simulink model "H250HILCtrl_400HzTypeXLOEUnknown"  (R2020b)
settings: Solver=FixedStepDiscrete  StartTime=0.0  StopTime=inf  FixedStep=Ts  RelTol=1e-3
InitFcn:
  | H250HILConInit_400HzTypeXLOEUnknown
values from neighbouring files (symbols this model uses):
  B = [0.25   -1.4142/(4*l)     1.4142/(4*l)     1/(4*c) ... (first row only)    [H250HILConInit_400HzTypeXLOEUnknown.m]
  g = (9.8)    (= 9.8)    [H250HILConInit_400HzTypeXLOEUnknown.m]
  J = (diag([0.0056 0.0056 0.0104]))    [H250HILConInit_400HzTypeXLOEUnknown.m]
  m = (0.752)    (= 0.752)    [H250HILConInit_400HzTypeXLOEUnknown.m]
  M = ([ 1          1          1         1 ... (first row only)    [H250HILConInit_400HzTypeXLOEUnknown.m]
  MY_ATT_P = Pixhawk_CSC.Parameter( {single(8), 'MY_ATT_P'}  )    [H250HILConInit_400HzTypeXLOEUnknown.m]
  MY_ATT_P_YAW = Pixhawk_CSC.Parameter( {single(0.0), 'MY_ATT_P_YAW'}  )    [H250HILConInit_400HzTypeXLOEUnknown.m]
  MY_POS_P = Pixhawk_CSC.Parameter( {single(0.6), 'MY_POS_P'}  )    [H250HILConInit_400HzTypeXLOEUnknown.m]
  MY_RATE_P = Pixhawk_CSC.Parameter( {single(12), 'MY_RATE_P'}  )    [H250HILConInit_400HzTypeXLOEUnknown.m]
  MY_RATE_P_YAW = Pixhawk_CSC.Parameter( {single(0.0), 'MY_RATE_P_YAW'}  )    [H250HILConInit_400HzTypeXLOEUnknown.m]
  MY_SAT_AD = Pixhawk_CSC.Parameter({single(0.13), 'MY_SAT_AD'} )    [H250HILConInit_400HzTypeXLOEUnknown.m]
  MY_TAU_P_A = Pixhawk_CSC.Parameter( {single(0.2), 'MY_TAU_P_A'}  )    [H250HILConInit_400HzTypeXLOEUnknown.m]
  MY_TAU_P_A_YAW = Pixhawk_CSC.Parameter( {single(0), 'MY_TAU_P_A_YAW'}  )    [H250HILConInit_400HzTypeXLOEUnknown.m]
  MY_TAU_P_P = Pixhawk_CSC.Parameter( {single(2.0), 'MY_TAU_P_P'}  )    [H250HILConInit_400HzTypeXLOEUnknown.m]
  MY_TAU_P_P_YAW = Pixhawk_CSC.Parameter( {single(0.04), 'MY_TAU_P_P_YAW'}  )    [H250HILConInit_400HzTypeXLOEUnknown.m]
  MY_VEL_P = Pixhawk_CSC.Parameter( {single(0.8), 'MY_VEL_P'}  )    [H250HILConInit_400HzTypeXLOEUnknown.m]
  T00 = single([m*g/4 m*g/4 m*g/4 m*g/4]')    [H250HILConInit_400HzTypeXLOEUnknown.m]
  Tf = 0.06    [H250HILConInit_400HzTypeXLOEUnknown.m]
  Tmotorbar = (0.032)    (= 0.032)    [H250HILConInit_400HzTypeXLOEUnknown.m]
  Ts = 1/400    (= 0.0025)    [H250HILConInit_400HzTypeXLOEUnknown.m]
libraries: discretizing x10, pixhawk_slib_uORB_RW x6, pixhawk_slib_sensors_actuators x5, pixhawk_slib_misc_utils x1, simulink x1, sharedtransform x1, pid_lib x1
(part 2 of 2)

== matlab function H250HILCtrl_400HzTypeXLOEUnknown/controller/innerloop/fmincon ==
  data: fd input; taop input; taoq input; taor input; T output; T0 input; M input; val output; time output
function [T,val,time] = fcn(fd, taop, taoq, taor, T0, M)
%% 求解
w1= 1;
w2 =20;
w3= 20;
w4= 0.00;
myfun2 = @(x)(w1*(M(1,:)*x-fd)^2+w2*(M(2,:)*x-taop)^2+w3*(M(3,:)*x-taoq)^2+w4*(M(4,:)*x-taor)^2);

lb  = [0 0 0 0]';
ub  = [3 3 3 3]';

options = optimoptions(@fmincon,'Algorithm','sqp','MaxIterations',10);
% tic
[T,val] = fmincon(myfun2,T0,[],[],[],[],lb,ub,[],options);
% ff = toc;
time =0;

== matlab function H250HILCtrl_400HzTypeXLOEUnknown/controller/innerloop/quadprog ==
  data: fd input double; taop input double; taoq input double; taor input double; T output double; T0 input double; M input double; fval output double; ub input double; iter output
function [T,fval, iter] = fcn(fd, taop, taoq, taor, T0, M, ub)
%% 求解
vd = [fd; taop; taoq; taor];
W=diag([1 20 20 0.01]);
H = M'*W*M;
f = -(vd'*W*M)';
% Td = B*vd;
lb  = [0 0 0 0]';
% ub  = [12 12 12 12]';
% if (max(B*vd)>3)||(min(B*vd)<0)
    options = optimoptions(@quadprog,'Algorithm','active-set','MaxIterations',10);

    [T,fval,~,output] = quadprog(H, f, [], [], [], [], lb, ub, T0, options);
     iter = output.iterations;
% else
%     T = B*vd;
%     fval = 0;
% end

== matlab function H250HILCtrl_400HzTypeXLOEUnknown/controller/innerloop/MATLAB Function1 ==
  data: u input; y output
function y = fcn(u)
y=diag([u,1,1,1]);

== matlab function H250HILCtrl_400HzTypeXLOEUnknown/controller/innerloop/MATLAB Function2 ==
  data: dT input; ub output
function ub = fcn(dT)
dub = zeros(4,1);
dub(1) = dT(1) - dT(3);
dub(2) = dT(2) - dT(4);
dub(3) = dT(3) - dT(1);
dub(4) = dT(4) - dT(2);
% dub(1) = dT(1);
% dub(2) = dT(2);
% dub(3) = dT(3);
% dub(4) = dT(4);
ub = [5 5 5 5]' + 1.8*min([dub(1) dub(2) dub(3) dub(4)]',[0 0 0 0]');%1.8

== matlab function H250HILCtrl_400HzTypeXLOEUnknown/controller/InputConditioning/MATLAB Function ==
  data: u input; y output
function y = fcn(u)

 if(u>1550)
    y=u;
 else
     if(u<1450)
     y=u;
     else
         y=single(1500);
     end
 end

== matlab function H250HILCtrl_400HzTypeXLOEUnknown/controller/InputConditioning/MATLAB Function1 ==
  data: u input; y output
function y = fcn(u)

 if(u>1550)
    y=u;
 else
     if(u<1450)
     y=u;
     else
         y=single(1500);
     end
 end

== matlab function H250HILCtrl_400HzTypeXLOEUnknown/controller/InputConditioning/MATLAB Function2 ==
  data: u input; y output
function y = fcn(u)

 if(u>1550)
    y=u;
 else
     if(u<1450)
     y=u;
     else
         y=single(1500);
     end
 end

== matlab function H250HILCtrl_400HzTypeXLOEUnknown/controller/quat2eul ==
  data: q input single; dcm output single
function dcm  = quat2eul(q)
% Conversion from Quaternion to Euler angles based on the PX4 Firmware
% v1.6.5 release.
% 
% Quaternion -> DCM -> Euler Angles
% INPUT:
%   q: Quaternion vector of the format: (a + bi + cj + dk)
% OUTPUT:
%   [phi,theta,psi]: Euler angles in radians.
% 
 if norm(q)~=0
    a = q(1);
    b = q(2);
    c = q(3);
    d = q(4);

    aSq = a*a;
    bSq = b*b;
    cSq = c*c;
    dSq = d*d;

    d_pi2 = pi/2;

    % quaternion_to_dcm
    dcm00 = aSq + bSq - cSq - dSq;
    dcm01 = 2*(b*c - a*d);
    dcm02 = 2*(a*c + b*d);
    dcm10 = 2*(b*c + a*d);
    dcm11 = aSq - bSq + cSq - dSq;
    dcm12 = 2*(c*d - a*b);
    dcm20 = 2*(b*d - a*c);
    dcm21 = 2*(a*b + c*d);
    dcm22 = aSq - bSq - cSq + dSq;
    dcm=[dcm00 dcm01 dcm02;
              dcm10 dcm11 dcm12;
              dcm20 dcm21  dcm22];
 else
     dcm = single(eye(3,3));
 end
    % dcm_to_euler

== matlab function H250HILCtrl_400HzTypeXLOEUnknown/controller/innerloop/Att ==
  data: e input; w input; psi input; pqrd output; ATT_P input; ATT_P_SCALE input
function pqrd  = fcn(e, w, psi, ATT_P, ATT_P_SCALE)
%% 角度控制1
% h1 = n3(1);
% h2 = n3(2);
% h3 = n3(3);
% h1d = n3d(1);
% h2d = n3d(2);
% h3d = n3d(3);
% we = Reb*w;
% k1 = single(5);
% epqd = [0 -1/h3; 1/h3 0]*[k1*(h1d-h1)+h2*we(3);k1*(h2d-h2)-h1*we(3)];
% 
% psid = single(0);
% rd = k1*0.3*(psid - psi);
% 
% Rbe = Reb';
% erd = (rd - Rbe(3,1)*epqd(1) - Rbe(3,2)*epqd(2))/Rbe(3,3);
% 
% pqd = Rbe((1:2),:)*[epqd; erd];%计算出机体系下的pqd
% pqd = mysat(pqd,2);
% pqrd = [pqd;rd];
%% 角度控制2
e1 = e(1);
e2 = e(2);
% e1  = n3(1) - n3d(1);
% e2  = n3(2) - n3d(2); 
beta = atan2(e2,e1);

k1 = ATT_P;
pqd = [ -k1*sqrt(e1^2+e2^2)*sin(psi-beta);
             -k1*sqrt(e1^2+e2^2)*cos(psi-beta);];
pqd = mysatsingle(pqd,3);
psid = 0;
% rd = -k1*0.3*(psi-psid);
rd = -k1*ATT_P_SCALE*(psi-psid);
% rd = 0;
pqrd = [pqd;rd];

== matlab function H250HILCtrl_400HzTypeXLOEUnknown/controller/Subsystem1/d_z ==
  data: n3 input size=[3,1]; dvz input single size=1; T_ input single size=4; M input single size=[4,4]; m input single size=1; g input single size=1; dz output single size=1
function dz   = fcn(n3, dvz, T_, M, m, g)
dz  = m*(dvz-g)/n3(3)+M(1,:)*T_;

== matlab function H250HILCtrl_400HzTypeXLOEUnknown/controller/Subsystem1/MATLAB Function2 ==
  data: throtte input; ad output; p input; v input; vhd input; POS_P input; VEL_P input
function ad = fcn(throtte, p, v, vhd, POS_P, VEL_P)
persistent pd
if isempty(pd)
    pd = single(p);
end
%% 高度通道
if throtte>=0.4&& throtte <=0.6
        vd3 = mysatsingle(POS_P * (pd(3) - p(3)), 0.5);
        ad3 = VEL_P * (vd3 - v(3));
else
    if throtte>0.6
        vd3 = -1;
        ad3 = VEL_P * (vd3 - v(3));
        pd(3) = p(3);
    else
        vd3 = 1;
        ad3 = VEL_P * (vd3 - v(3));
        pd(3) = p(3);
    end
end
%% 水平通道
if norm(vhd) <= 0.05
        vd12 = mysatsingle(POS_P * (pd(1:2) - p(1:2)), 0.5);
        ad12 = VEL_P * (vd12 - v(1:2));
else
        vd12 = mysatsingle(5*vhd, 0.7);
        ad12 = VEL_P * (vd12 - v(1:2));
        pd(1:2) = p(1:2);
end
ad = [ad12;ad3];

== matlab function H250HILCtrl_400HzTypeXLOEUnknown/controller/Subsystem2/MATLAB Function ==
  data: Reb input; psi output
function psi = fcn(Reb)
psi = atan2(Reb(2,1), Reb(1,1));

== matlab function H250HILCtrl_400HzTypeXLOEUnknown/controller/Subsystem1/Pos ==
  data: ad3 input single size=[3,1]; n3 input; m input single size=1; fd output single size=1; g input single size=1; n3d output single size=3; ad output single size=3; SAT_AD input
function [fd, n3d, ad]  = fcn(ad3, n3, m, g, SAT_AD)
 

% ad3 = [ad1(1)+ad2(1); ad1(2)+ad2(2); ad1(3)+ad2(3)];

ad = mysatsingle(ad3,single(SAT_AD)*g);

n3d = ([single(0); single(0); g]-ad)/norm([single(0); single(0); g]-ad);
if n3d(3)==single(0)
    fd = single(0);
else
    fd = m*(g-ad(3))/n3(3);
%     fd = m*g-ad(3);
end
